simulink subsystem "MixSamples"  (R2024a)
settings: Solver=VariableStepAuto  StartTime=0.0  StopTime=10.0  RelTol=1e-3
undefined symbols (not defined in the file or in its folder): max_midi_data
settings Model: Creator=david  LastModifiedBy=david

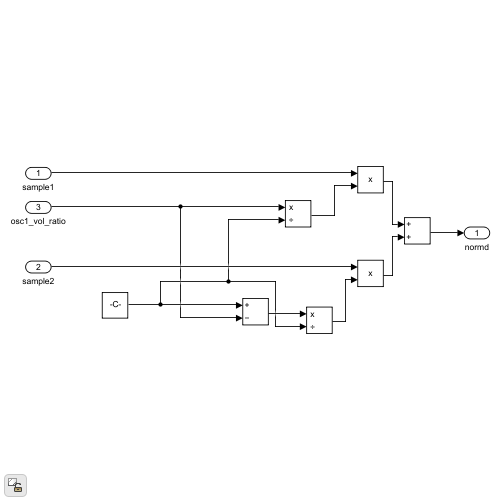
[thumbnail: Simulink's stored preview of the top-level diagram]
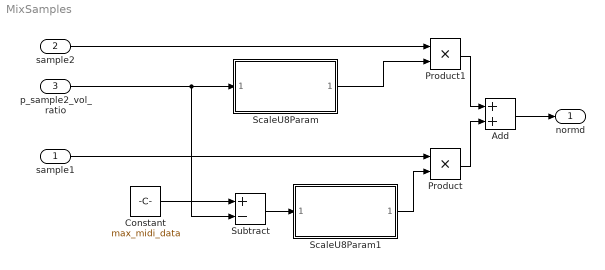
== system MixSamples ==
  sample1 : Inport
  sample2 : Inport  Port=2
  p_sample2_vol_ratio : Inport  Port=3
  Add : Sum
  Constant : Constant  Value=max_midi_data
  Product : Product
  Product1 : Product
  ScaleU8Param : Subsystem  ReferencedSubsystem=ScaleU8Param
  ScaleU8Param1 : Subsystem  ReferencedSubsystem=ScaleU8Param
  Subtract : Sum  Inputs=+-
  normd : Outport
  wires:
  sample1/1 -> Product/1
  Product/1 -> Add/2
  Constant/1 -> Subtract/1
  ScaleU8Param1/1 -> Product/2
  Product1/1 -> Add/1
  ScaleU8Param/1 -> Product1/2
  sample2/1 -> Product1/1
  Add/1 -> normd/1
  p_sample2_vol_ratio/1 -> Subtract/2, ScaleU8Param/1
  Subtract/1 -> ScaleU8Param1/1
